simulink model "DC_Motor_Model"  (R2024b)
settings: Solver=FixedStepAuto  StartTime=0.0  StopTime=10.0  FixedStep=1e-4  RelTol=1e-3
undefined symbols (not defined in the file or in its folder): B, J, Kb, Kt, L, R
settings Model: Creator=Nabil  LastModifiedBy=Nabil

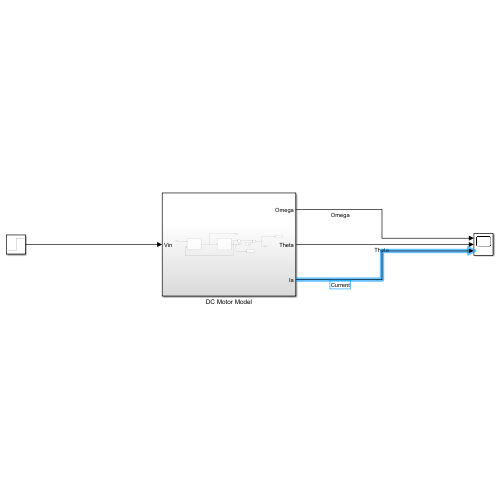
[thumbnail: Simulink's stored preview of the top-level diagram]
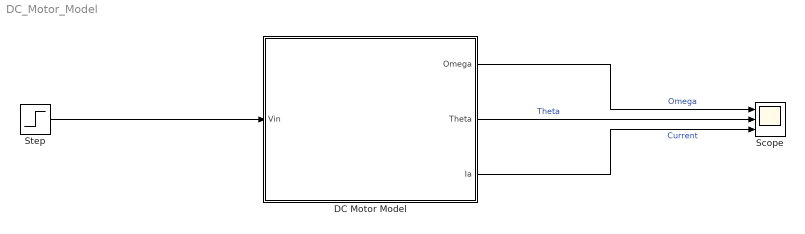
== system DC_Motor_Model ==
  DC Motor Model : Subsystem
  Scope : Scope  NumInputPorts=3
  Step : Step  SampleTime=0
  wires:
  Step/1 -> DC Motor Model/1(Vin)
  DC Motor Model/1(Omega) -> Scope/1  "Omega"
  DC Motor Model/2(Theta) -> Scope/2  "Theta"
  DC Motor Model/3(Ia) -> Scope/3  "Current"

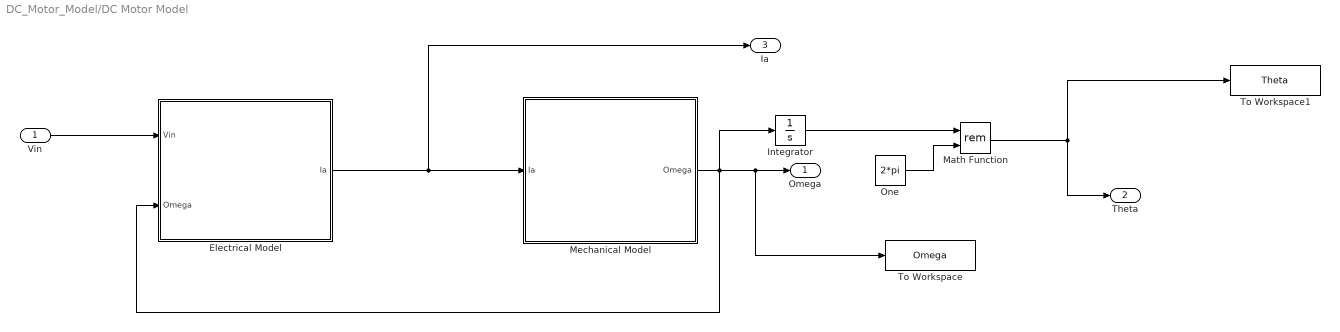
== system DC_Motor_Model/DC Motor Model ==
  Vin : Inport
  Electrical Model : Subsystem
  Integrator : Integrator  WrappedStateUpperValue=2*pi  WrappedStateLowerValue=0
  Math Function : Math  Operator=rem
  Mechanical Model : Subsystem
  One : Constant  Value=2*pi  OutDataTypeStr=Inherit: Inherit via back propagation
  To Workspace : ToWorkspace  VariableName=Omega  SaveFormat=Timeseries  SampleTime=-1
  To Workspace1 : ToWorkspace  VariableName=Theta  SaveFormat=Timeseries  SampleTime=-1
  Omega : Outport
  Theta : Outport  Port=2
  Ia : Outport  Port=3
  wires:
  Vin/1 -> Electrical Model/1(Vin)
  Mechanical Model/1(Omega) -> To Workspace/1, Omega/1, Integrator/1, Electrical Model/2(Omega)
  Electrical Model/1(Ia) -> Ia/1, Mechanical Model/1(Ia)
  Integrator/1 -> Math Function/1
  Math Function/1 -> Theta/1, To Workspace1/1
  One/1 -> Math Function/2

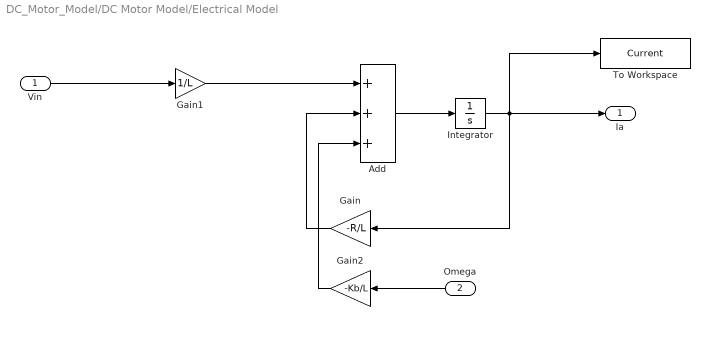
== system DC_Motor_Model/DC Motor Model/Electrical Model ==
  Vin : Inport
  Omega : Inport  Port=2
  Add : Sum  Inputs=+++
  Gain : Gain  Gain=-R/L
  Gain1 : Gain  Gain=1/L
  Gain2 : Gain  Gain=-Kb/L
  Integrator : Integrator
  To Workspace : ToWorkspace  VariableName=Current  SaveFormat=Timeseries  SampleTime=-1
  Ia : Outport
  wires:
  Add/1 -> Integrator/1
  Vin/1 -> Gain1/1
  Integrator/1 -> Ia/1, Gain/1, To Workspace/1
  Omega/1 -> Gain2/1
  Gain/1 -> Add/2
  Gain1/1 -> Add/1
  Gain2/1 -> Add/3

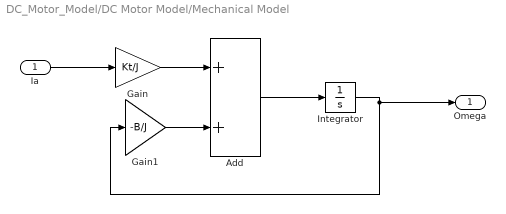
== system DC_Motor_Model/DC Motor Model/Mechanical Model ==
  Ia : Inport
  Add : Sum
  Gain : Gain  Gain=Kt/J
  Gain1 : Gain  Gain=-B/J
  Integrator : Integrator
  Omega : Outport
  wires:
  Integrator/1 -> Omega/1, Gain1/1
  Gain1/1 -> Add/2
  Gain/1 -> Add/1
  Ia/1 -> Gain/1
  Add/1 -> Integrator/1
